simulink model "BallAndBeamModel_v1_velocity"  (R2022b)
settings: Solver=VariableStepAuto  StartTime=0.0  StopTime=1.5  RelTol=1e-3
libraries: simulink x1
settings Model: Creator=andre  LastModifiedBy=andre

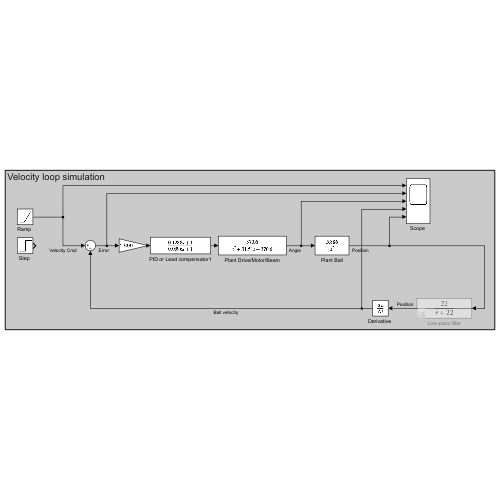
[thumbnail: Simulink's stored preview of the top-level diagram]
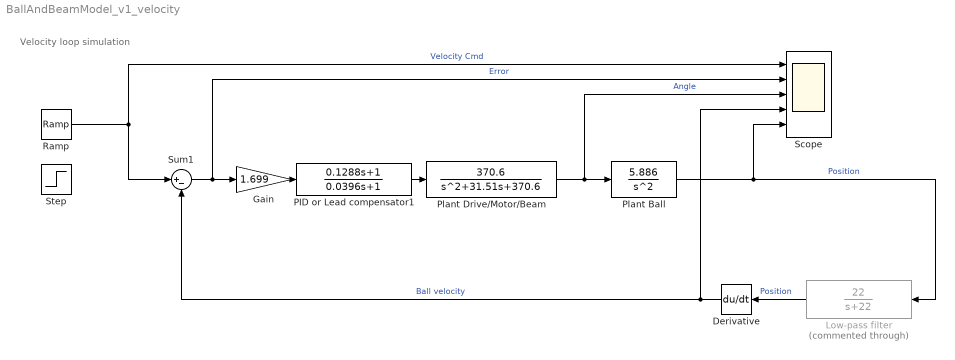
== system BallAndBeamModel_v1_velocity ==
  note: Velocity loop simulation
  "Derivative " : Derivative
  Gain : Gain  Gain=1.699
  Low-pass filter : TransferFcn  Commented=through  Numerator=[ 22]  Denominator=[1 22]
  PID or Lead compensator1 : TransferFcn  Numerator=[0.1288 1]  Denominator=[0.0396 1]
  Plant Ball : TransferFcn  Numerator=[5.886]  Denominator=[1 0 0]
  Plant Drive/Motor/Beam : TransferFcn  Numerator=[370.6]  Denominator=[1 31.51 370.6]
  "Ramp " : simulink/Sources/Ramp  slope=1  start=0  InitialOutput=0
  "Scope " : Scope  NumInputPorts=5
  "Step " : Step  Time=0.1  After=0.1  SampleTime=0
  Sum1 : Sum  Inputs=|+-
  wires:
  Low-pass filter/1 -> "Derivative "/1  "Position"
  Plant Drive/Motor/Beam/1 -> "Scope "/3, Plant Ball/1  "Angle"
  "Derivative "/1 -> "Scope "/4, Sum1/2  "Ball velocity"
  Sum1/1 -> "Scope "/2, Gain/1  "Error"
  PID or Lead compensator1/1 -> Plant Drive/Motor/Beam/1
  Gain/1 -> PID or Lead compensator1/1
  "Ramp "/1 -> Sum1/1, "Scope "/1  "Velocity Cmd"
  Plant Ball/1 -> "Scope "/5, Low-pass filter/1  "Position"
